simulink library "honestlibrary"  (R2013b)
settings: Solver=ode45  StartTime=0.0  StopTime=10.0  RelTol=1e-3
libraries: honestlibrary x192, xbsIndex_r4 x32
(part 2 of 2)

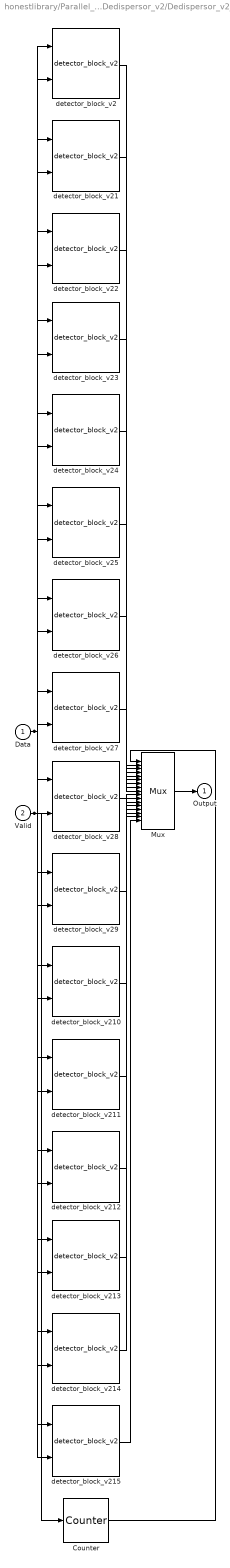
== system honestlibrary/Parallel_Dedispersor_v2/Dedispersor_v2_2 ==
  Data : Inport
  Valid : Inport  Port=2
  Counter : xbsIndex_r4/Counter  cnt_type=Free Running  cnt_to=Inf  operation=Up  start_count=0  cnt_by_val=1  arith_type=Unsigned  n_bits=4  bin_pt=0  load_pin=off  rst=off  en=on  explicit_period=on  period=1  dbl_ovrd=off  use_behavioral_HDL=off  implementation=Fabric  block_type=counter
  Mux : xbsIndex_r4/Mux  inputs=16  en=off  latency=0  precision=Full  arith_type=Unsigned  n_bits=16  bin_pt=14  quantization=Truncate  overflow=Wrap  dbl_ovrd=off  block_type=mux
  detector_block_v2 : honestlibrary/detector_block_v2  chn=0  lat=1  nbits=4
      settings: AttributesFormatString=Channel: 4, Delay: 9
  detector_block_v21 : honestlibrary/detector_block_v2  chn=1  lat=2  nbits=4
      settings: AttributesFormatString=Channel: 4, Delay: 9
  detector_block_v210 : honestlibrary/detector_block_v2  chn=10  lat=11  nbits=4
      settings: AttributesFormatString=Channel: 4, Delay: 9
  detector_block_v211 : honestlibrary/detector_block_v2  chn=11  lat=12  nbits=4
      settings: AttributesFormatString=Channel: 4, Delay: 9
  detector_block_v212 : honestlibrary/detector_block_v2  chn=12  lat=13  nbits=4
      settings: AttributesFormatString=Channel: 4, Delay: 9
  detector_block_v213 : honestlibrary/detector_block_v2  chn=13  lat=14  nbits=4
      settings: AttributesFormatString=Channel: 4, Delay: 9
  detector_block_v214 : honestlibrary/detector_block_v2  chn=14  lat=15  nbits=4
      settings: AttributesFormatString=Channel: 4, Delay: 9
  detector_block_v215 : honestlibrary/detector_block_v2  chn=15  lat=16  nbits=4
      settings: AttributesFormatString=Channel: 4, Delay: 9
  detector_block_v22 : honestlibrary/detector_block_v2  chn=2  lat=3  nbits=4
      settings: AttributesFormatString=Channel: 4, Delay: 9
  detector_block_v23 : honestlibrary/detector_block_v2  chn=3  lat=4  nbits=4
      settings: AttributesFormatString=Channel: 4, Delay: 9
  detector_block_v24 : honestlibrary/detector_block_v2  chn=4  lat=5  nbits=4
      settings: AttributesFormatString=Channel: 4, Delay: 9
  detector_block_v25 : honestlibrary/detector_block_v2  chn=5  lat=6  nbits=4
      settings: AttributesFormatString=Channel: 4, Delay: 9
  detector_block_v26 : honestlibrary/detector_block_v2  chn=6  lat=7  nbits=4
      settings: AttributesFormatString=Channel: 4, Delay: 9
  detector_block_v27 : honestlibrary/detector_block_v2  chn=7  lat=8  nbits=4
      settings: AttributesFormatString=Channel: 4, Delay: 9
  detector_block_v28 : honestlibrary/detector_block_v2  chn=8  lat=9  nbits=4
      settings: AttributesFormatString=Channel: 4, Delay: 9
  detector_block_v29 : honestlibrary/detector_block_v2  chn=9  lat=10  nbits=4
      settings: AttributesFormatString=Channel: 4, Delay: 9
  Output : Outport
  wires:
  Counter/1 -> Mux/1
  detector_block_v2/1 -> Mux/2
  detector_block_v21/1 -> Mux/3
  detector_block_v22/1 -> Mux/4
  detector_block_v23/1 -> Mux/5
  detector_block_v24/1 -> Mux/6
  detector_block_v25/1 -> Mux/7
  detector_block_v26/1 -> Mux/8
  detector_block_v27/1 -> Mux/9
  detector_block_v28/1 -> Mux/10
  detector_block_v29/1 -> Mux/11
  detector_block_v210/1 -> Mux/12
  detector_block_v211/1 -> Mux/13
  detector_block_v212/1 -> Mux/14
  detector_block_v213/1 -> Mux/15
  detector_block_v214/1 -> Mux/16
  detector_block_v215/1 -> Mux/17
  Mux/1 -> Output/1
  Valid/1 -> detector_block_v2/2, detector_block_v21/2, detector_block_v22/2, detector_block_v23/2, detector_block_v24/2, detector_block_v25/2, detector_block_v26/2, detector_block_v27/2, detector_block_v28/2, detector_block_v29/2, detector_block_v210/2, detector_block_v211/2, detector_block_v212/2, detector_block_v213/2, detector_block_v214/2, detector_block_v215/2, Counter/1
  Data/1 -> detector_block_v2/1, detector_block_v21/1, detector_block_v22/1, detector_block_v23/1, detector_block_v24/1, detector_block_v25/1, detector_block_v26/1, detector_block_v27/1, detector_block_v28/1, detector_block_v29/1, detector_block_v210/1, detector_block_v211/1, detector_block_v212/1, detector_block_v213/1, detector_block_v214/1, detector_block_v215/1

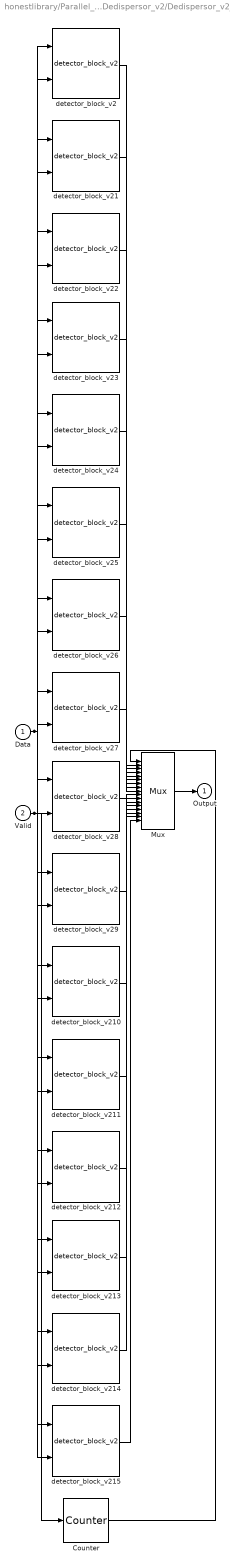
== system honestlibrary/Parallel_Dedispersor_v2/Dedispersor_v2_3 ==
  Data : Inport
  Valid : Inport  Port=2
  Counter : xbsIndex_r4/Counter  cnt_type=Free Running  cnt_to=Inf  operation=Up  start_count=0  cnt_by_val=1  arith_type=Unsigned  n_bits=4  bin_pt=0  load_pin=off  rst=off  en=on  explicit_period=on  period=1  dbl_ovrd=off  use_behavioral_HDL=off  implementation=Fabric  block_type=counter
  Mux : xbsIndex_r4/Mux  inputs=16  en=off  latency=0  precision=Full  arith_type=Unsigned  n_bits=16  bin_pt=14  quantization=Truncate  overflow=Wrap  dbl_ovrd=off  block_type=mux
  detector_block_v2 : honestlibrary/detector_block_v2  chn=0  lat=1  nbits=4
      settings: AttributesFormatString=Channel: 4, Delay: 9
  detector_block_v21 : honestlibrary/detector_block_v2  chn=1  lat=2  nbits=4
      settings: AttributesFormatString=Channel: 4, Delay: 9
  detector_block_v210 : honestlibrary/detector_block_v2  chn=10  lat=11  nbits=4
      settings: AttributesFormatString=Channel: 4, Delay: 9
  detector_block_v211 : honestlibrary/detector_block_v2  chn=11  lat=12  nbits=4
      settings: AttributesFormatString=Channel: 4, Delay: 9
  detector_block_v212 : honestlibrary/detector_block_v2  chn=12  lat=13  nbits=4
      settings: AttributesFormatString=Channel: 4, Delay: 9
  detector_block_v213 : honestlibrary/detector_block_v2  chn=13  lat=14  nbits=4
      settings: AttributesFormatString=Channel: 4, Delay: 9
  detector_block_v214 : honestlibrary/detector_block_v2  chn=14  lat=15  nbits=4
      settings: AttributesFormatString=Channel: 4, Delay: 9
  detector_block_v215 : honestlibrary/detector_block_v2  chn=15  lat=16  nbits=4
      settings: AttributesFormatString=Channel: 4, Delay: 9
  detector_block_v22 : honestlibrary/detector_block_v2  chn=2  lat=3  nbits=4
      settings: AttributesFormatString=Channel: 4, Delay: 9
  detector_block_v23 : honestlibrary/detector_block_v2  chn=3  lat=4  nbits=4
      settings: AttributesFormatString=Channel: 4, Delay: 9
  detector_block_v24 : honestlibrary/detector_block_v2  chn=4  lat=5  nbits=4
      settings: AttributesFormatString=Channel: 4, Delay: 9
  detector_block_v25 : honestlibrary/detector_block_v2  chn=5  lat=6  nbits=4
      settings: AttributesFormatString=Channel: 4, Delay: 9
  detector_block_v26 : honestlibrary/detector_block_v2  chn=6  lat=7  nbits=4
      settings: AttributesFormatString=Channel: 4, Delay: 9
  detector_block_v27 : honestlibrary/detector_block_v2  chn=7  lat=8  nbits=4
      settings: AttributesFormatString=Channel: 4, Delay: 9
  detector_block_v28 : honestlibrary/detector_block_v2  chn=8  lat=9  nbits=4
      settings: AttributesFormatString=Channel: 4, Delay: 9
  detector_block_v29 : honestlibrary/detector_block_v2  chn=9  lat=10  nbits=4
      settings: AttributesFormatString=Channel: 4, Delay: 9
  Output : Outport
  wires:
  Counter/1 -> Mux/1
  detector_block_v2/1 -> Mux/2
  detector_block_v21/1 -> Mux/3
  detector_block_v22/1 -> Mux/4
  detector_block_v23/1 -> Mux/5
  detector_block_v24/1 -> Mux/6
  detector_block_v25/1 -> Mux/7
  detector_block_v26/1 -> Mux/8
  detector_block_v27/1 -> Mux/9
  detector_block_v28/1 -> Mux/10
  detector_block_v29/1 -> Mux/11
  detector_block_v210/1 -> Mux/12
  detector_block_v211/1 -> Mux/13
  detector_block_v212/1 -> Mux/14
  detector_block_v213/1 -> Mux/15
  detector_block_v214/1 -> Mux/16
  detector_block_v215/1 -> Mux/17
  Mux/1 -> Output/1
  Valid/1 -> detector_block_v2/2, detector_block_v21/2, detector_block_v22/2, detector_block_v23/2, detector_block_v24/2, detector_block_v25/2, detector_block_v26/2, detector_block_v27/2, detector_block_v28/2, detector_block_v29/2, detector_block_v210/2, detector_block_v211/2, detector_block_v212/2, detector_block_v213/2, detector_block_v214/2, detector_block_v215/2, Counter/1
  Data/1 -> detector_block_v2/1, detector_block_v21/1, detector_block_v22/1, detector_block_v23/1, detector_block_v24/1, detector_block_v25/1, detector_block_v26/1, detector_block_v27/1, detector_block_v28/1, detector_block_v29/1, detector_block_v210/1, detector_block_v211/1, detector_block_v212/1, detector_block_v213/1, detector_block_v214/1, detector_block_v215/1

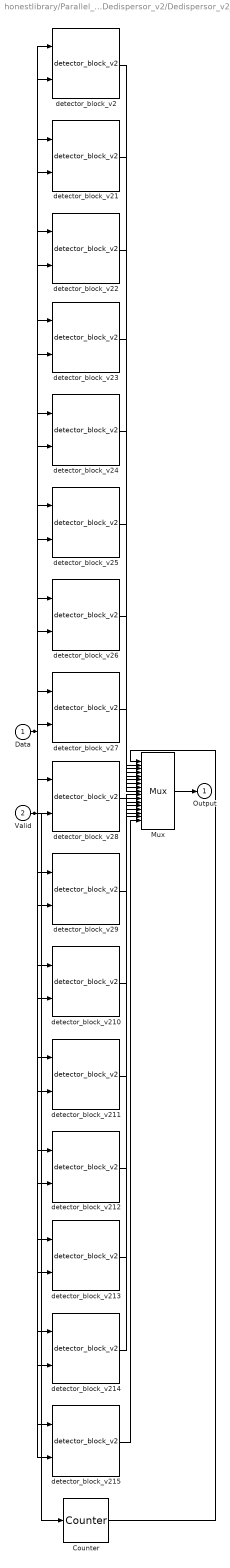
== system honestlibrary/Parallel_Dedispersor_v2/Dedispersor_v2_4 ==
  Data : Inport
  Valid : Inport  Port=2
  Counter : xbsIndex_r4/Counter  cnt_type=Free Running  cnt_to=Inf  operation=Up  start_count=0  cnt_by_val=1  arith_type=Unsigned  n_bits=4  bin_pt=0  load_pin=off  rst=off  en=on  explicit_period=on  period=1  dbl_ovrd=off  use_behavioral_HDL=off  implementation=Fabric  block_type=counter
  Mux : xbsIndex_r4/Mux  inputs=16  en=off  latency=0  precision=Full  arith_type=Unsigned  n_bits=16  bin_pt=14  quantization=Truncate  overflow=Wrap  dbl_ovrd=off  block_type=mux
  detector_block_v2 : honestlibrary/detector_block_v2  chn=0  lat=1  nbits=4
      settings: AttributesFormatString=Channel: 4, Delay: 9
  detector_block_v21 : honestlibrary/detector_block_v2  chn=1  lat=2  nbits=4
      settings: AttributesFormatString=Channel: 4, Delay: 9
  detector_block_v210 : honestlibrary/detector_block_v2  chn=10  lat=11  nbits=4
      settings: AttributesFormatString=Channel: 4, Delay: 9
  detector_block_v211 : honestlibrary/detector_block_v2  chn=11  lat=12  nbits=4
      settings: AttributesFormatString=Channel: 4, Delay: 9
  detector_block_v212 : honestlibrary/detector_block_v2  chn=12  lat=13  nbits=4
      settings: AttributesFormatString=Channel: 4, Delay: 9
  detector_block_v213 : honestlibrary/detector_block_v2  chn=13  lat=14  nbits=4
      settings: AttributesFormatString=Channel: 4, Delay: 9
  detector_block_v214 : honestlibrary/detector_block_v2  chn=14  lat=15  nbits=4
      settings: AttributesFormatString=Channel: 4, Delay: 9
  detector_block_v215 : honestlibrary/detector_block_v2  chn=15  lat=16  nbits=4
      settings: AttributesFormatString=Channel: 4, Delay: 9
  detector_block_v22 : honestlibrary/detector_block_v2  chn=2  lat=3  nbits=4
      settings: AttributesFormatString=Channel: 4, Delay: 9
  detector_block_v23 : honestlibrary/detector_block_v2  chn=3  lat=4  nbits=4
      settings: AttributesFormatString=Channel: 4, Delay: 9
  detector_block_v24 : honestlibrary/detector_block_v2  chn=4  lat=5  nbits=4
      settings: AttributesFormatString=Channel: 4, Delay: 9
  detector_block_v25 : honestlibrary/detector_block_v2  chn=5  lat=6  nbits=4
      settings: AttributesFormatString=Channel: 4, Delay: 9
  detector_block_v26 : honestlibrary/detector_block_v2  chn=6  lat=7  nbits=4
      settings: AttributesFormatString=Channel: 4, Delay: 9
  detector_block_v27 : honestlibrary/detector_block_v2  chn=7  lat=8  nbits=4
      settings: AttributesFormatString=Channel: 4, Delay: 9
  detector_block_v28 : honestlibrary/detector_block_v2  chn=8  lat=9  nbits=4
      settings: AttributesFormatString=Channel: 4, Delay: 9
  detector_block_v29 : honestlibrary/detector_block_v2  chn=9  lat=10  nbits=4
      settings: AttributesFormatString=Channel: 4, Delay: 9
  Output : Outport
  wires:
  Counter/1 -> Mux/1
  detector_block_v2/1 -> Mux/2
  detector_block_v21/1 -> Mux/3
  detector_block_v22/1 -> Mux/4
  detector_block_v23/1 -> Mux/5
  detector_block_v24/1 -> Mux/6
  detector_block_v25/1 -> Mux/7
  detector_block_v26/1 -> Mux/8
  detector_block_v27/1 -> Mux/9
  detector_block_v28/1 -> Mux/10
  detector_block_v29/1 -> Mux/11
  detector_block_v210/1 -> Mux/12
  detector_block_v211/1 -> Mux/13
  detector_block_v212/1 -> Mux/14
  detector_block_v213/1 -> Mux/15
  detector_block_v214/1 -> Mux/16
  detector_block_v215/1 -> Mux/17
  Mux/1 -> Output/1
  Valid/1 -> detector_block_v2/2, detector_block_v21/2, detector_block_v22/2, detector_block_v23/2, detector_block_v24/2, detector_block_v25/2, detector_block_v26/2, detector_block_v27/2, detector_block_v28/2, detector_block_v29/2, detector_block_v210/2, detector_block_v211/2, detector_block_v212/2, detector_block_v213/2, detector_block_v214/2, detector_block_v215/2, Counter/1
  Data/1 -> detector_block_v2/1, detector_block_v21/1, detector_block_v22/1, detector_block_v23/1, detector_block_v24/1, detector_block_v25/1, detector_block_v26/1, detector_block_v27/1, detector_block_v28/1, detector_block_v29/1, detector_block_v210/1, detector_block_v211/1, detector_block_v212/1, detector_block_v213/1, detector_block_v214/1, detector_block_v215/1
